simulink subsystem "uav_plant_subsystem"  (R2025a)
settings: Solver=VariableStepAuto  StartTime=0.0  StopTime=10.0  RelTol=1e-3
values from neighbouring files (symbols this model uses):
  ini_position = [0;10]    [actual_uav_parameters_xflr5.m]
  ini_velocity = [15;0]    [actual_uav_parameters_xflr5.m]
  Mass = 2.02    [actual_uav_parameters_xflr5.m]
settings Model: Creator=Zyad  LastModifiedBy=Zyad

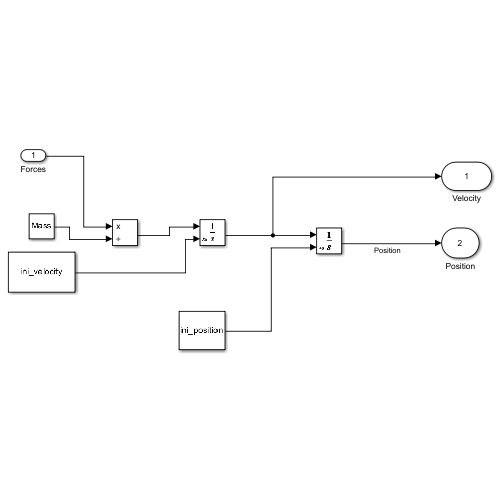
[thumbnail: Simulink's stored preview of the top-level diagram]
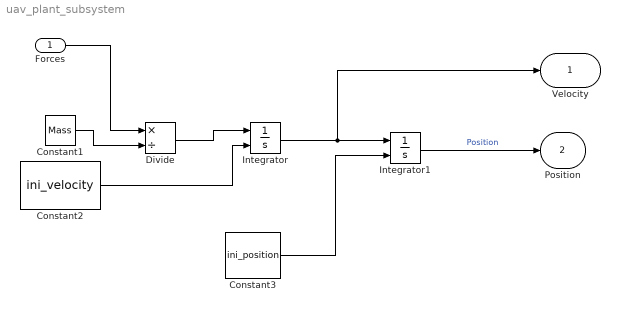
== system uav_plant_subsystem ==
  Forces : Inport
  Constant1 : Constant  Value=Mass
  Constant2 : Constant  Value=ini_velocity
  Constant3 : Constant  Value=ini_position
  Divide : Product  Inputs=*/
  Integrator : Integrator  InitialConditionSource=external
  Integrator1 : Integrator  InitialConditionSource=external
  Velocity : Outport
  Position : Outport  Port=2
  wires:
  Forces/1 -> Divide/1
  Constant1/1 -> Divide/2
  Divide/1 -> Integrator/1
  Constant2/1 -> Integrator/2
  Integrator/1 -> Velocity/1, Integrator1/1
  Constant3/1 -> Integrator1/2
  Integrator1/1 -> Position/1  "Position"
